simulink model "problem1_model"  (R2023b)
settings: Solver=VariableStepAuto  StartTime=0.0  StopTime=200  RelTol=1e-3
values from neighbouring files (symbols this model uses):
  h = 2    [Project.m]
  k = 2    [Project.m]
  M_2 = 1    [Project.m]
  M_3 = 0.5    [Project.m]
  S_1 = 0.5    [Project.m]
  S_2 = 1    [Project.m]
settings Model: Creator=afons  LastModifiedBy=afons

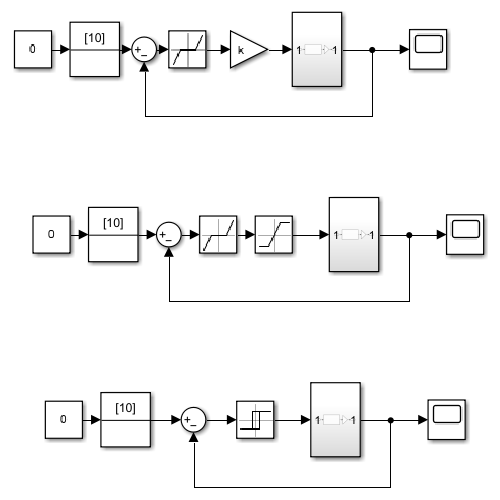
[thumbnail: Simulink's stored preview of the top-level diagram]
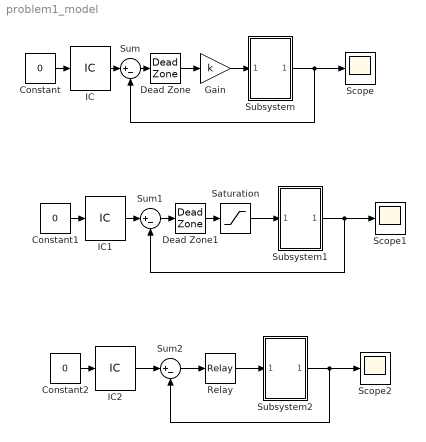
== system problem1_model ==
  Constant : Constant  Value=0
  Constant1 : Constant  Value=0
  Constant2 : Constant  Value=0
  Dead Zone : DeadZone  LowerValue=-S_1  UpperValue=S_1
  Dead Zone1 : DeadZone  LowerValue=-S_2  UpperValue=S_2
  Gain : Gain  Gain=k
  IC : InitialCondition  Value=10
  IC1 : InitialCondition  Value=10
  IC2 : InitialCondition  Value=10
  Relay : Relay  OnSwitchValue=h  OffSwitchValue=-h  OnOutputValue=M_3  OffOutputValue=-M_3
  Saturation : Saturate  UpperLimit=M_2  LowerLimit=-M_2
  Scope : Scope
  Scope1 : Scope
  Scope2 : Scope
  Subsystem : Subsystem
  Subsystem1 : Subsystem
  Subsystem2 : Subsystem
  Sum : Sum  Inputs=|+-
  Sum1 : Sum  Inputs=|+-
  Sum2 : Sum  Inputs=|+-
  wires:
  Dead Zone1/1 -> Saturation/1
  Sum/1 -> Dead Zone/1
  Subsystem/1(Out1) -> Sum/2, Scope/1
  IC1/1 -> Sum1/1
  Subsystem1/1(Out1) -> Sum1/2, Scope1/1
  Saturation/1 -> Subsystem1/1(In1)
  Sum1/1 -> Dead Zone1/1
  IC2/1 -> Sum2/1
  Subsystem2/1(Out1) -> Sum2/2, Scope2/1
  Relay/1 -> Subsystem2/1(In1)
  Sum2/1 -> Relay/1
  Dead Zone/1 -> Gain/1
  Gain/1 -> Subsystem/1(In1)
  Constant/1 -> IC/1
  IC/1 -> Sum/1
  Constant1/1 -> IC1/1
  Constant2/1 -> IC2/1

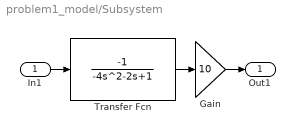
== system problem1_model/Subsystem ==
  In1 : Inport
  Gain : Gain  Gain=10
  Transfer Fcn : TransferFcn  Numerator=[-1]  Denominator=[-4 , -2 , 1]
  Out1 : Outport
  wires:
  Transfer Fcn/1 -> Gain/1
  In1/1 -> Transfer Fcn/1
  Gain/1 -> Out1/1

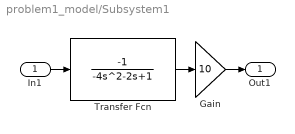
== system problem1_model/Subsystem1 ==
  In1 : Inport
  Gain : Gain  Gain=10
  Transfer Fcn : TransferFcn  Numerator=[-1]  Denominator=[-4 , -2 , 1]
  Out1 : Outport
  wires:
  Transfer Fcn/1 -> Gain/1
  In1/1 -> Transfer Fcn/1
  Gain/1 -> Out1/1

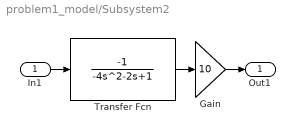
== system problem1_model/Subsystem2 ==
  In1 : Inport
  Gain : Gain  Gain=10
  Transfer Fcn : TransferFcn  Numerator=[-1]  Denominator=[-4 , -2 , 1]
  Out1 : Outport
  wires:
  Transfer Fcn/1 -> Gain/1
  In1/1 -> Transfer Fcn/1
  Gain/1 -> Out1/1
